simulink model "control_att_lqr"  (R2020a)
settings: Solver=FixedStepAuto  StartTime=0.0  StopTime=10.0  FixedStep=1/simVars.freq  RelTol=1e-3
undefined symbols (not defined in the file or in its folder): par
libraries: simulink x1, eeGeneralControl x1
settings Model: Creator=LocalAdmin  LastModifiedBy=sihao
settings DataIOCC: SaveOutput=off  SaveTime=off
settings OptimizationCC: DefaultParameterBehavior=Inlined
settings HardwareCC: ProdBitPerPointer=32  ProdBitPerSizeT=32  ProdBitPerPtrDiffT=32  ProdLargestAtomicFloat=None  ProdWordSize=32  ProdLongLongMode=on  ProdHWDeviceType=Custom Processor->Custom Processor
settings SFSimCC: CustomCodeUndefinedFunction=UseInterfaceOnly
settings RTWCC: TargetLang=C++
settings GRTTargetCC: TargetLangStandard=C++03 (ISO)  CombineOutputUpdateFcns=off  MatFileLogging=off  SupportVariableSizeSignals=on

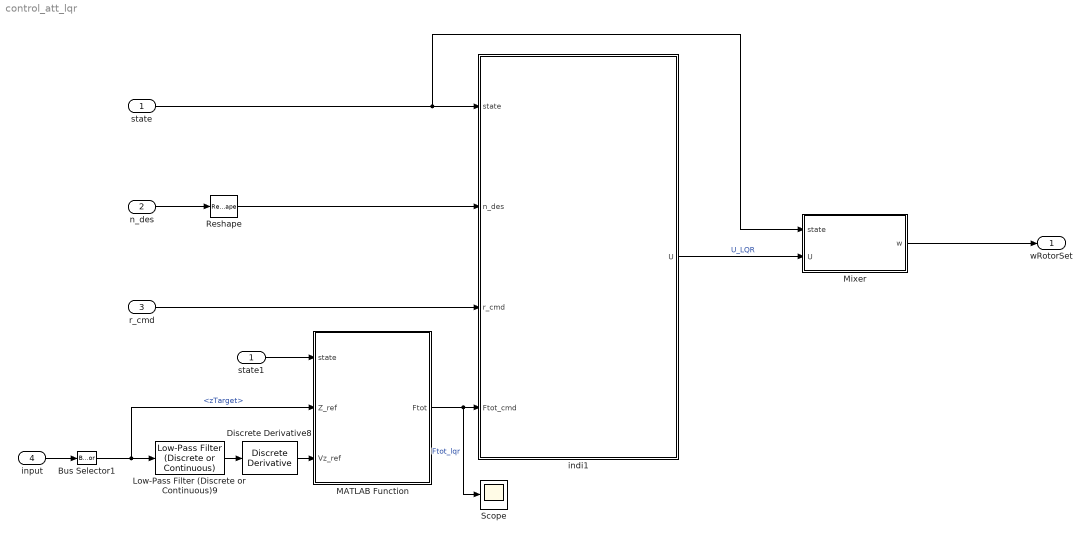
== system control_att_lqr ==
  state : Inport  OutDataTypeStr=Bus: stateBus
  n_des : Inport  Port=2
  r_cmd : Inport  Port=3
  input : Inport  Port=4  OutDataTypeStr=Bus: inputsBus
  Bus Selector1 : BusSelector  OutputSignals=zTarget
  Discrete Derivative8 : simulink/Discrete/Discrete Derivative  gainval=1.0  ICPrevScaledInput=0.0  OutMin=[]  OutMax=[]  OutDataType=fixdt(1, 16)  OutScaling=2^-10  DoSatur=off
  Low-Pass Filter (Discrete or Continuous)9 : eeGeneralControl/Low-Pass Filter (Discrete or Continuous)  K=1  T=par.t_indi  B=inf  A=-inf  init_option=Inherited from block input  x0=0  Ts=-1
  MATLAB Function : MATLAB Function  TreatAsAtomicUnit=on
  Mixer : MATLAB Function  TreatAsAtomicUnit=on
  Reshape : Reshape
  Scope : Scope
  indi1 : MATLAB Function  TreatAsAtomicUnit=on
  state1 : InportShadow  OutDataTypeStr=Bus: stateBus
  wRotorSet : Outport  SignalName=wRotorSet  VectorParamsAs1DForOutWhenUnconnected=off
  wires:
  indi1/1(U) -> Mixer/2(U)  "U_LQR"
  Mixer/1(w) -> wRotorSet/1
  state/1 -> Mixer/1(state), indi1/1(state)
  n_des/1 -> Reshape/1
  Reshape/1 -> indi1/2(n_des)
  r_cmd/1 -> indi1/3(r_cmd)
  MATLAB Function/1(Ftot) -> Scope/1, indi1/4(Ftot_cmd)  "Ftot_lqr"
  state1/1 -> MATLAB Function/1(state)
  Low-Pass Filter (Discrete or Continuous)9/1 -> Discrete Derivative8/1
  Bus Selector1/1 -> Low-Pass Filter (Discrete or Continuous)9/1, MATLAB Function/2(Z_ref)  "<zTarget>"
  Discrete Derivative8/1 -> MATLAB Function/3(Vz_ref)
  input/1 -> Bus Selector1/1

== matlab function control_att_lqr/MATLAB Function ==
  data: state input; Z_ref input; Ftot output; Vz_ref input; par parameter
function Ftot = calcFtot(state,Z_ref, Vz_ref, par)
    Ftot = calcFtot(state,Z_ref, Vz_ref, par);
end

== matlab function control_att_lqr/Mixer ==
  data: state input Bus: stateBus; U input; w output size=[4,1]; par parameter
function w = Mixer(state, U, par)
% U = [s * k0 * (w4^2 - w2^2); 
%      s * k0 * (w1^2 - w3^2); 
%      k0 * (w1^2 + w2^2 + w3^2 + w4^2);
%      t0 * (w1^2 - w2^2 + w3^2 - w4^2)]
% w: rotor speed commands


if par.DRF_enable && state.fail_id > 0
    if state.fail_id == 1 || state.fail_id == 3
        fail_id = [1 3];
    else %if state.fail_id == 2 || state.fail_id == 4
        fail_id = [2 4];
    end
else
    fail_id = state.fail_id;
end

w = zeros(4,1);

s = par.lqr.s;
k0 = par.k0;
t0 = par.t0;
% mass = par.mass;

G0 = [0 -1 0 1;
     1 0 -1 0;
     1 1 1 1;
     1 -1 1 -1];
 
G = diag([s*k0, s*k0, k0, t0])*G0;
if sum(fail_id)>0 
    G(:,fail_id) = zeros(4,length(fail_id));
end

w2 = pinv(G)*U;

% if length(state.fail_id) == 2  
%     w2(1) = (U(1) + U(3))/2;
%     w2(2) = 0;
%     w2(3) = (-U(1) + U(3))/2;
%     w2(4) = 0;    
% elseif length(state.fail_id) == 1
%     G(
%     w2(1) = (U(1) - U(2) + U(3))/2;
%     w2(2) = U(2);
%     w2(3) = (-U(1) - U(2) + U(3))/2;
%     w2(4) = 0;
% else 
%     w2 =  [0        0.5000    0.2500    0.2500
%           -0.5000   0         0.2500    -0.2500
%            0       -0.5000    0.2500    0.2500
%            0.5000   0         0.2500    -0.2500] * [U(3);U(1);U(2);U(4)];
% end
w(1) = sqrt(abs(w2(1)))*sign(w2(1));
w(2) = sqrt(abs(w2(2)))*sign(w2(2));
w(3) = sqrt(abs(w2(3)))*sign(w2(3));
w(4) = sqrt(abs(w2(4)))*sign(w2(4));

w(w<par.w_min) = par.w_min;
w(w>par.w_max) = par.w_max;

end

== matlab function control_att_lqr/indi1 ==
  data: state input Bus: stateBus; U output; n_des input size=[3,1]; r_cmd input; Ftot_cmd input; par parameter
function U   = control_reduced_att_lqr(state,n_des,r_cmd,Ftot_cmd, par)

[U] = control_reduced_att_lqr(state,n_des,Ftot_cmd, r_cmd, par);

end
